simulink model "simpleprocess_vector"  (Simulink 7.4)
settings: Solver=ode45  StartTime=0.0  StopTime=10.0  RelTol=1e-3
undefined symbols (not defined in the file or in its folder): A, B, C
settings Model: Creator=Alex  LastModifiedBy=Alex

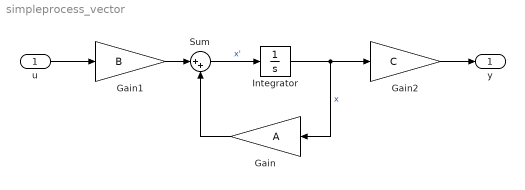
== system simpleprocess_vector ==
  u : Inport  OutDataType=fixdt(1, 16)  OutScaling=2^0
  Gain : Gain  Gain=A  ParameterDataType=fixdt(1, 16)  ParameterScaling=2^0  OutDataType=fixdt(1, 16)  OutScaling=2^0
  Gain1 : Gain  Gain=B  ParameterDataType=fixdt(1, 16)  ParameterScaling=2^0  OutDataType=fixdt(1, 16)  OutScaling=2^0
  Gain2 : Gain  Gain=C  ParameterDataType=fixdt(1, 16)  ParameterScaling=2^0  OutDataType=fixdt(1, 16)  OutScaling=2^0
  Integrator : Integrator
  Sum : Sum  Inputs=|++  OutDataType=fixdt(1, 16)  OutScaling=2^0
  y : Outport  OutDataType=fixdt(1, 16)  OutScaling=2^0
  wires:
  Gain/1 -> Sum/2
  Sum/1 -> Integrator/1  "x'"
  Integrator/1 -> Gain2/1, Gain/1  "x"
  Gain1/1 -> Sum/1
  Gain2/1 -> y/1
  u/1 -> Gain1/1
